simulink model "testbench_or_control"  (R2016a)
settings: Solver=FixedStepAuto  StartTime=0.0  StopTime=10.0  RelTol=1e-3
libraries: legoev3lib x5
settings Model: SimulationMode=external  ExtModeTrigDuration=2  Creator=Shobhit  LastModifiedBy=Shobhit
settings SolverCC: PositivePriorityOrder=on
settings OptimizationCC: OptimizeModelRefInitCode=on  LifeSpan=1  MaxStackSize=64
settings HardwareCC: ProdBitPerPointer=32  ProdLargestAtomicInteger=Long  ProdWordSize=32  ProdHWDeviceType=ARM Compatible->ARM 9  UseEmbeddedCoderFeatures=off  UseSimulinkCoderFeatures=off
settings RTWCC: SystemTargetFile=ert.tlc  HardwareBoard=LEGO MINDSTORMS EV3  TemplateMakefile=ert_default_tmf  GenerateReport=on  Toolchain=Sourcery G++ Lite v2009q3  IncludeHyperlinkInReport=on  LaunchReport=on  GenerateTraceInfo=on  GenerateTraceReport=on  GenerateTraceReportSl=on  GenerateTraceReportSf=on  GenerateTraceReportEml=on
settings CodeAppCC: ForceParamTrailComments=on  IgnoreCustomStorageClasses=off  OperatorAnnotations=on  SimulinkDataObjDesc=on  SFDataObjDesc=on  MATLABFcnDesc=on  InsertBlockDesc=on  MATLABSourceComments=on
settings ERTTargetCC: SupportContinuousTime=on  SupportNonInlinedSFcns=on  SupportVariableSizeSignals=on

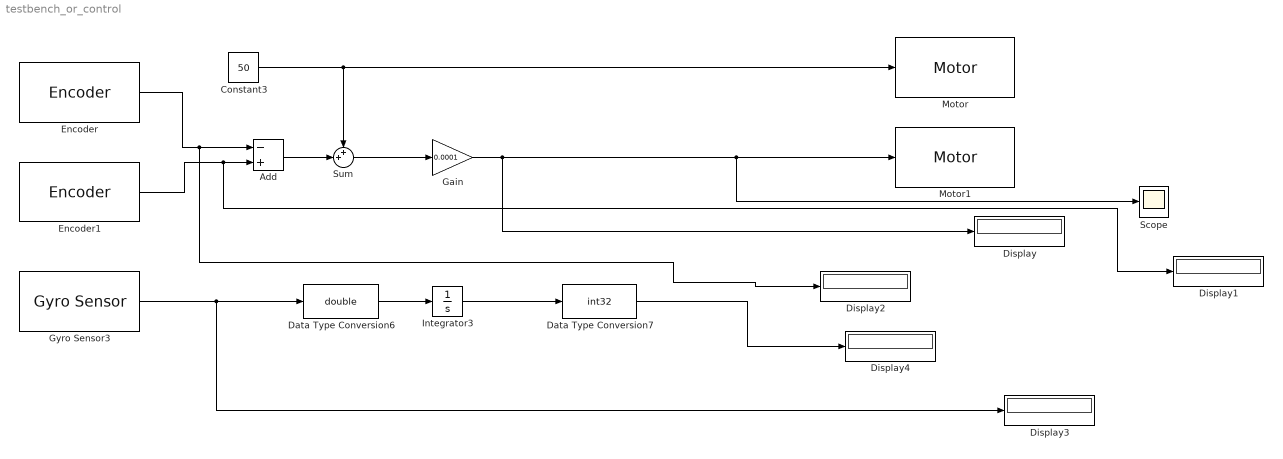
== system testbench_or_control ==
  Add : Sum  Inputs=-+
  Constant3 : Constant  Value=50
  Data Type Conversion6 : DataTypeConversion  OutDataTypeStr=double  RndMeth=Ceiling
  Data Type Conversion7 : DataTypeConversion  OutDataTypeStr=int32  RndMeth=Ceiling
  Display{,1..4} (5 alike) : Display
      Display4 settings: Format=decimal (Stored Integer)
  Encoder : legoev3lib/Encoder  portNumber=A  opMode=Reset at each sample time  sampleTime=0.1
  Encoder1 : legoev3lib/Encoder  portNumber=B  opMode=No reset  sampleTime=0.1
  Gain : Gain  Gain=0.0001
  Gyro Sensor3 : legoev3lib/Gyro Sensor  portNumber=2  sampleTime=0.1
  Integrator3 : Integrator
  Motor : legoev3lib/Motor  sportNumber=A  sstopAction=Brake
  Motor1 : legoev3lib/Motor  sportNumber=B  sstopAction=Brake
  Scope : Scope
  Sum : Sum  Inputs=++|
  wires:
  Constant3/1 -> Sum/1, Motor/1
  Encoder1/1 -> Display1/1, Add/2
  Add/1 -> Sum/2
  Sum/1 -> Gain/1
  Gain/1 -> Display/1, Motor1/1, Scope/1
  Integrator3/1 -> Data Type Conversion7/1
  Data Type Conversion6/1 -> Integrator3/1
  Encoder/1 -> Display2/1, Add/1
  Gyro Sensor3/1 -> Display3/1, Data Type Conversion6/1
  Data Type Conversion7/1 -> Display4/1
